simulink model "sf_backup_undesirable"  (R2017b)
settings: Solver=FixedStepDiscrete  StartTime=0.0  StopTime=1  FixedStep=.2  RelTol=1e-3  EnableMultiTasking=on
settings Model: Creator=The MathWorks, Inc.  LastModifiedBy=The MathWorks, Inc.
settings DataIOCC: LimitDataPoints=on  SaveFormat=Array
settings OptimizationCC: ExpressionDepthLimit=2147483647  InitFltsAndDblsToZero=on  LifeSpan=inf
settings DebuggingCC: SaveWithParameterizedLinksMsg=none  UnderspecifiedInitializationDetection=Classic  MergeDetectMultiDrivingBlocksExec=none  SignalResolutionControl=TryResolveAllWithWarning  SolverPrmCheckMsg=warning  MultiTaskDSMMsg=warning  MultiTaskCondExecSysMsg=none  FcnCallInpInsideContextMsg=warning  StateNameClashWarn=warning  StrictBusMsg=Warning  SFUnexpectedBacktrackingDiag=warning  SFNoUnconditionalDefaultTransitionDiag=warning  SFExecutionAtInitializationDiag=none
settings HardwareCC: ProdBitPerPointer=32  ProdBitPerSizeT=32  ProdBitPerPtrDiffT=32  ProdLargestAtomicFloat=None  ProdIntDivRoundTo=Undefined  ProdEndianess=Unspecified  ProdWordSize=32  ProdHWDeviceType=32-bit Generic
settings ModelReferenceCC: PropagateSignalLabelsOutOfModel=off
settings SFSimCC: SimParseCustomCode=off
settings CodeAppCC: StateflowObjectComments=on
settings GRTTargetCC: TargetFcnLib=ansi_tfl_tmw.mat  TargetLangStandard=C89/C90 (ANSI)  GeneratePreprocessorConditionals=Disable all  CombineOutputUpdateFcns=off  GRTInterface=on
settings ConfigComp: CovMetricSettings=dw  CovHtmlReporting=on  CovSaveCumulativeToWorkspaceVar=on  CovSaveSingleToWorkspaceVar=on  CovExternalEMLEnable=off  CovSFcnEnable=off

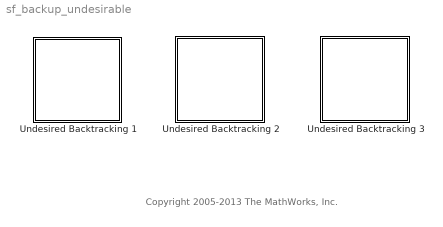
== system sf_backup_undesirable ==
  note: Copyright 2005-2013 The MathWorks, Inc.
  Undesired Backtracking 1 : Stateflow chart  TreatAsAtomicUnit=on
  Undesired Backtracking 2 : Stateflow chart  TreatAsAtomicUnit=on
      settings: RTWFcnNameOpts=Use subsystem name  RTWFileNameOpts=Use subsystem name
  Undesired Backtracking 3 : Stateflow chart  TreatAsAtomicUnit=on
      settings: RTWFcnNameOpts=Use subsystem name  RTWFileNameOpts=Use subsystem name

== stateflow chart sf_backup_undesirable/Undesired Backtracking 3 ==
  settings: updateMethod=DISCRETE  executeAtInitialization=1
  state BAD [function]
    note: The function BAD shows an example of backtracking which can lead to
        | inefficient run-time behavior. A cursory examination of the flowgraph
        | to the right might lead one to believe that it represents the following
        | run-time behavior:
        |
        | if ( (foo1() || foo2()) &&
        |       (foo3() || foo4()) &&
        |       (foo5() || foo6()) &&
        |       foo7() ) {
        |         action();
        | }
        |
        | Suppose that all the functions fooN return true EXCEPT foo7. In this case,
        | the backtracking semantics will lead to multiple calls to some of the functions.
        | For example, the function foo5() might get called upto 4 times. The more the
        | number of these "stages", the higher the computational cost.
        |
        | In addition to the runtime cost, the generated code will also tend to bloat due
        | to multiple copies of the flow graph code.
    (default) -> (junction 45)
    (junction 45) -> (junction 46) [order 1] : [foo1()]
    (junction 45) -> (junction 46) [order 2] : [foo2()]
    (junction 46) -> (junction 47) [order 1] : [foo3()]
    (junction 46) -> (junction 47) [order 2] : [foo4()]
    (junction 47) -> (junction 48) [order 2] : [foo6()]
    (junction 47) -> (junction 48) [order 1] : [foo5()]
    (junction 48) -> (junction 50) : [foo7()]
        | {action();}
  state GOOD [function]
    note: The function GOOD shows a way in which you can obtain the runtime
        | semantics below, while still achieving good computation and code generation
        | efficiency. By providing default paths to terminal junctions, the generated
        | code actually resembles the pseudo code below:
        |
        | if ( (foo1() || foo2()) &&
        |       (foo3() || foo4()) &&
        |       (foo5() || foo6()) &&
        |       foo7() ) {
        |         action();
        | }
        |
        | Therefore it is easy to see that in the case that all the functions fooN except
        | foo7 return true, the functions foo1(), foo3(), foo5() and foo7() will get called
        | exactly once rather than multiple times.
    (default) -> (junction 58)
    (junction 58) -> (junction 59) [order 1] : [foo1()]
    (junction 58) -> (junction 59) [order 2] : [foo2()]
    (junction 59) -> (junction 73) [order 3]
    (junction 59) -> (junction 60) [order 1] : [foo3()]
    (junction 59) -> (junction 60) [order 2] : [foo4()]
    (junction 60) -> (junction 75) [order 3]
    (junction 60) -> (junction 61) [order 2] : [foo6()]
    (junction 60) -> (junction 61) [order 1] : [foo5()]
    (junction 61) -> (junction 77) [order 2]
    (junction 61) -> (junction 62) [order 1] : [foo7()]
        | {action();}

== stateflow chart sf_backup_undesirable/Undesired Backtracking 1 ==
  state BAD [function]
    note: The function 'BAD' shows an example of backtracking semantics
        | which may not be expected or desired. When conditions c1, c2
        | and c3 are true but c4 is false, the backtracking semantics
        | results in multiple executions of the condition action 'a3++'.
        |
        | 1. c1 is checked and is true
        | 2. Therefore c3 is checked. It is true, therfore 'a3++' is execued
        | 3. c4 is then checked. It is false. Now execution backtracks to the
        | last junction which still has unchecked transitions. In this case,
        | we backtrack to c2.
        | 4. c2 is checked and is true.
        | 5. c3 is checked again. Again it is true and 'a3++' is repeated again!
        | 6. c4 is checked and it is false. This time there are no transitions
        | to backtrack to. So execution stops.
    (default) -> (junction 38)
    (junction 38) -> (junction 39) [order 1] : [c1]
    (junction 38) -> (junction 39) [order 2] : [c2]
    (junction 39) -> (junction 43) : [c3]{a3++;}
    (junction 43) -> (junction 45) : [c4]
  state GOOD [function]
    note: In contrast, in this function, there are no junctions which have
        | multiple paths leading to them. This prevents us from backtracking
        | and hence the action 'a3++' is executed exactly once.
        |
        | Notice that the semantics of GOOD and BAD are quite different.
    (default) -> (junction 48)
    (junction 48) -> (junction 49) : [c1 || c2]
    (junction 49) -> (junction 50) : [c3]{a3++;}
    (junction 50) -> (junction 51) : [c4]
  data: a1 local double; a2 local double; a3 local double; a4 local double; a5 local double; a6 local double; a7 local double; c1 local double =1; c2 local double; c3 local double =0; c4 local double; c5 local double; c6 local double; c7 local double

== stateflow chart sf_backup_undesirable/Undesired Backtracking 2 ==
  settings: updateMethod=DISCRETE  executeAtInitialization=1
  state BAD [function]
    note: The function BAD shows an example of backtracking semantics which
        | may not be expected or desired. A cursory look at the flow graph might
        | lead one to believe that it represents the following pseudo code:
        |
        | if (u1) {
        |     if_u1_true;
        | } else {
        |     if _u1_false;
        | }
        |
        | if (u2) {
        |      if_u2_true;
        | }
        |
        | However, in the case when u1 is true but u2 is false, both the actions
        | if_u1_true and if_u1_false are executed! This is because of backtracking
        | semantics. When control reaches u2 for the first time (along if_u1_true) and it
        | evaluates to false, we backtrack to if_u1_false because it was not previously
        | checked. This leads to if_u1_false also getting executed.
    (default) -> (junction 9)
    (junction 9) -> (junction 14) [order 1] : [u1]
    (junction 14) -> (junction 15) : {if_u1_true;}
    (junction 9) -> (junction 10) [order 2] : {if_u1_false;}
    (junction 15) -> (junction 10)
    (junction 10) -> (junction 11)
    (junction 11) -> (junction 13) : [u2]
    (junction 13) -> (junction 12) : {if_u2_true;}
  state GOOD [function]
    note: The function GOOD shows how to avoid the problem with undesired
        | backtracking. The correct way to do it is to add a default transition to
        | a terminal junction. This prevents us from backtracking from u2 all
        | the way to if_u2_false. Instead, as soon as u2 is tried and is found to
        | be false, the execution flows to the terminal junction and stops. This
        | means that we get the semantics shown in the pseudo code above.
    (default) -> (junction 23)
    (junction 23) -> (junction 24) [order 1] : [u1]
    (junction 24) -> (junction 26) : {if_u1_true;}
    (junction 23) -> (junction 25) [order 2] : {if_u1_false;}
    (junction 26) -> (junction 25)
    (junction 25) -> (junction 27)
    (junction 27) -> (junction 28) [order 1] : [u2]
    (junction 27) -> (junction 40) [order 2]
    (junction 28) -> (junction 29) : {if_u2_true;}
